simulink model "zynqRadioHWSWQPSKAD9361AD9364SL_UDP_SourceSelect"  (R2016a)
settings: Solver=FixedStepAuto  StartTime=0.0  StopTime=1  RelTol=1e-3
libraries: dspnetwork x1
settings Model: Creator=The MathWorks, Inc.  LastModifiedBy=The MathWorks, Inc.

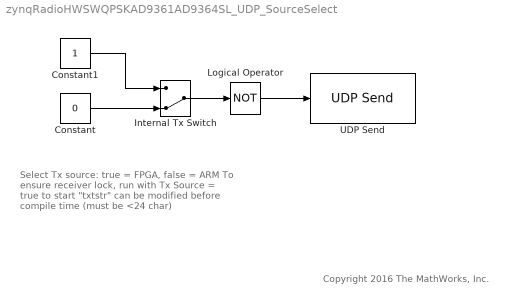
== system zynqRadioHWSWQPSKAD9361AD9364SL_UDP_SourceSelect ==
  note: Select Tx source:
      | true = FPGA, false = ARM
      |
      | To ensure receiver lock, run with Tx
      | Source = true to start
      |
      | "txtstr" can be modified before
      | compile time (must be <24 char)
  note: Copyright 2016 The MathWorks, Inc.
  Constant : Constant  Value=0  OutDataTypeStr=boolean  SampleTime=-1
  Constant1 : Constant  OutDataTypeStr=boolean  SampleTime=1
  Internal Tx Switch : ManualSwitch  CurrentSetting=0
  Logical Operator : Logic  Operator=NOT  AllPortsSameDT=off  OutDataTypeStr=boolean
  UDP Send : dspnetwork/UDP Send  remoteURL='192.168.3.2'  remotePort=25000  localURL='0.0.0.0'  localPortSource=Automatically determine  localPort=-1  sampletime=-1  separateLengthPort=0
  wires:
  Constant/1 -> Internal Tx Switch/2
  Constant1/1 -> Internal Tx Switch/1
  Internal Tx Switch/1 -> Logical Operator/1
  Logical Operator/1 -> UDP Send/1
